simulink model "two_channel"  (R2022b)
settings: Solver=FixedStepAuto  StartTime=0.0  StopTime=3  FixedStep=1/fs  RelTol=1e-3
libraries: spsSecondOrderFilterLib x2
settings Model: Creator=joaovitor  LastModifiedBy=joaovitor

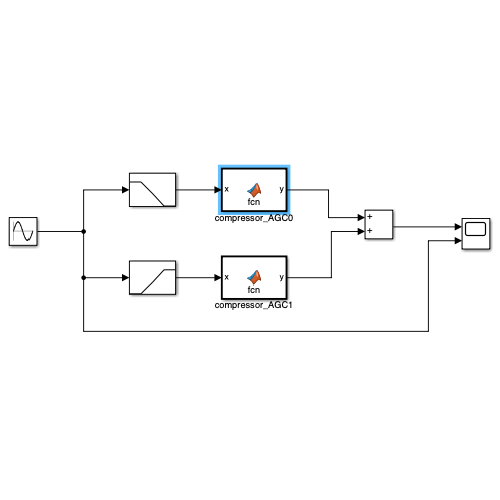
[thumbnail: Simulink's stored preview of the top-level diagram]
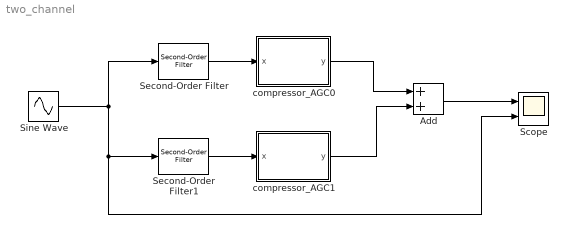
== system two_channel ==
  Add : Sum
  Scope : Scope  NumInputPorts=2
  Second-Order Filter : spsSecondOrderFilterLib/Second-Order Filter  FilterType=Lowpass  Fo=2800  Zeta=0.707  Ts=0  Initialize=on  Vac_Init="[0,  0,  60]"  Vdc_Init=0  PlotResponse=off  FreqRange=[0, 500, 1]
      settings: LibrarySourceBlock=|
      | sps_lib/Control/Filters/Second-Order
      | Filter
  Second-Order Filter1 : spsSecondOrderFilterLib/Second-Order Filter  FilterType=Highpass  Fo=2800  Zeta=0.707  Ts=0  Initialize=on  Vac_Init="[0,  0,  60]"  Vdc_Init=0  PlotResponse=off  FreqRange=[0, 500, 1]
      settings: LibrarySourceBlock=|
      | sps_lib/Control/Filters/Second-Order
      | Filter
  Sine Wave : Sin  Frequency=44*2*pi  SampleTime=0
  compressor_AGC0 : MATLAB Function  TreatAsAtomicUnit=on
  compressor_AGC1 : MATLAB Function  TreatAsAtomicUnit=on
  wires:
  Second-Order Filter/1 -> compressor_AGC0/1(x)
  Second-Order Filter1/1 -> compressor_AGC1/1(x)
  compressor_AGC0/1(y) -> Add/1
  compressor_AGC1/1(y) -> Add/2
  Add/1 -> Scope/1
  Sine Wave/1 -> Second-Order Filter1/1, Scope/2, Second-Order Filter/1

== matlab function two_channel/compressor_AGC1 ==
  data: x input; y output
function y = fcn(x)
    % Call the custom function defined in the same directory
    threshold = -10;       % Example threshold value
    ratio = 2;             % Example compression ratio
    fs = 1000;             % Sampling frequency
    attack_time = 0.1;     % Attack time in seconds
    release_time = 0.2;    % Release time in seconds

    y = compressor_AGC(x, threshold, ratio, fs, attack_time, release_time);
end

== matlab function two_channel/compressor_AGC0 ==
  data: x input; y output
function y = fcn(x)
    % Call the custom function defined in the same directory
    threshold = -10;       % Example threshold value
    ratio = 2;             % Example compression ratio
    fs = 1000;             % Sampling frequency
    attack_time = 0.1;     % Attack time in seconds
    release_time = 0.2;    % Release time in seconds

    y = compressor_AGC(x, threshold, ratio, fs, attack_time, release_time);
end
